simulink model "EX_display_2"  (Simulink 4.00)
settings: Solver=ode45  StartTime=0.0  StopTime=10.0  RelTol=1e-3
settings Model: LastModifiedBy=Администратор

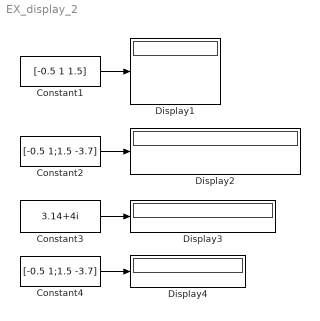
== system EX_display_2 ==
  Constant1 : Constant  Value=[-0.5 1 1.5]
  Constant2 : Constant  Value=[-0.5 1;1.5 -3.7]  VectorParams1D=off
  Constant3 : Constant  Value=3.14+4i
  Constant4 : Constant  Value=[-0.5 1;1.5 -3.7]  VectorParams1D=off
  Display{1..4} (4 alike) : Display
      settings: Format=short
  wires:
  Constant1/1 -> Display1/1
  Constant2/1 -> Display2/1
  Constant3/1 -> Display3/1
  Constant4/1 -> Display4/1
